simulink library "pbbs_final"  (Simulink 8.1)
settings: Solver=ode1  StartTime=0.0  StopTime=Inf  FixedStep=0.001  RelTol=1e-3
PostLoadFcn:
  | , if any(exist('dsrtsu_mdlpostloadfcn', 'file') == [2, 3, 6]), try dsrtsu_mdlpostloadfcn('Execute', bdroot); catch fprintf('Error in PostLoadFcn (dsrtsu_mdlpostloadfcn) for model "%s":\n %s\n', bdroot, lasterr); end, end,
undefined symbols (not defined in the file or in its folder): KJUD_DecelHardBraking_mps2, KJUD_DecelTGapBraking_s, KJUD_SDFDelay_s, ZERO_FLOAT
libraries: hcu_lib x1, ebdc x1, frdc x1
settings Model: DSRTSU_INTERNAL_RTI_VER=450  DSRTSU_INTERNAL_RTI_TYPE=rti1401  RTICANMMDATA=struct('GeneralSetupData',struct('modelroot','D:\ELN150201\Phase3\branches\ACC_Experiments\AdasDragon\software\sw_development\arch\app\jud','generalsettings',struct('filesettings',struct('destfolder',struct('Name','RTICANMM_FILES','Check',1),'buildfolder',struct('Name','.','Check',1),'AbsDestfolder',struct('Name','D:\ELN150201\Phase3\branches\ACC_Experiments\AdasDragon\software\sw_development\arch\app\jud\RTICANMM_FILES'),'AbsBuildfolder',struct('Name','D:\ELN150201\Phase3\branches\ACC_Experiments\AdasDragon\software\sw_development\arch\app\jud'))),'options',struct('addpaths',1,'rmpaths',1,'addtrcexclusion',logical(1),'cannavigator',struct('checkmonitoring',0),'show_usrtrc',0,'use_usrtrc',0),'advanced',struct('options',[1 1 1 1 1 1 1 1 1 1 1 1 1 1 1 1 1 1 1 1 1 1 1 1 1 1 1 1 1 1 1 1 1 1 1 1 1 1 1 1 1 1 1 1 1 1 1 1 1 1 1 1 1 1 1 1 1 1 1 1 1 1 1 1 1 1 1 1 1 1 1 1 1 1 1 1 1 1 1 1 1 1 1 1 1 1 1 1 1 1 1 1 1 1 1 1 1 1 1 1]),'MPSetup',{{}},'modelname','pbbs_final','block','pbbs_final'))  DSRTSU_INTERNAL_RTIFPGA=40  Creator=tescamilla  LastModifiedBy=AT015555

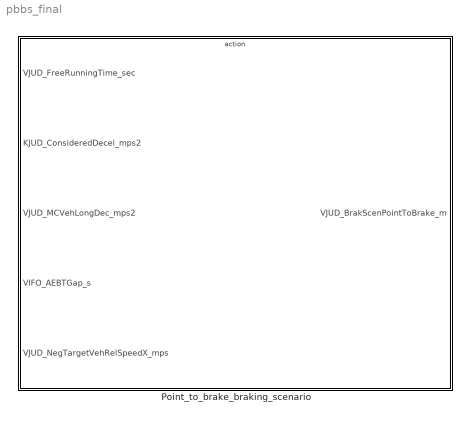
== system pbbs_final ==
  Point_to_brake_braking_scenario : Subsystem

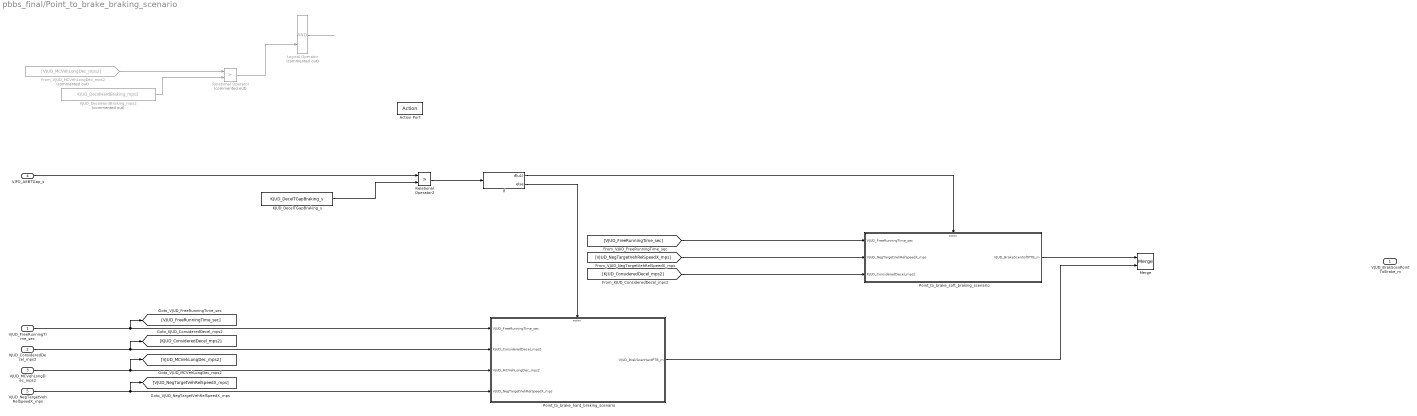
== system pbbs_final/Point_to_brake_braking_scenario ==
  VJUD_FreeRunningTime_sec : Inport
  KJUD_ConsideredDecel_mps2 : Inport  Port=2
  VJUD_MCVehLongDec_mps2 : Inport  Port=3
  VIFO_AEBTGap_s : Inport  Port=4
  VJUD_NegTargetVehRelSpeedX_mps : Inport  Port=5
  Action Port : ActionPort
  From_VJUD_MCVehLongDec_mps2 : From  Commented=on  GotoTag=VJUD_MCVehLongDec_mps2
  If : If  IfExpression=u1
  KJUD_DecelHardBraking_mps2 : Constant  Commented=on  Value=KJUD_DecelHardBraking_mps2  OutDataTypeStr=single
  KJUD_DecelTGapBraking_s : Constant  Value=KJUD_DecelTGapBraking_s  OutDataTypeStr=single
  Logical Operator : Logic  Commented=on  AllPortsSameDT=off  OutDataTypeStr=boolean
  Merge : Merge
  Point_to_brake_hard_braking_scenario : Subsystem  TreatAsAtomicUnit=on
  Point_to_brake_soft_braking_scenario : Subsystem
  Relational Operator : RelationalOperator  Commented=on  Operator=>  OutDataTypeStr=boolean
  Relational Operator2 : RelationalOperator  Operator=>  OutDataTypeStr=boolean
  VJUD_BrakScenPointToBrake_m : Outport
  wires:
  ? -> VJUD_BrakScenPointToBrake_m/1  "VJUD_BrakScenPointToBrake_m"
  [VJUD_NegTargetVehRelSpeedX_mps] -> Point_to_brake_soft_braking_scenario/2(VJUD_NegTargetVehRelSpeedX_mps)
  [KJUD_ConsideredDecel_mps2] -> Point_to_brake_soft_braking_scenario/3(KJUD_ConsideredDecel_mps2)
  [VJUD_FreeRunningTime_sec] -> Point_to_brake_soft_braking_scenario/1(VJUD_FreeRunningTime_sec)
  Point_to_brake_hard_braking_scenario/1(VJUD_BrakScenHardPTB_m) -> Merge/2
  Point_to_brake_soft_braking_scenario/1(VJUD_BrakeScenSoftPTB_m) -> Merge/1
  VJUD_MCVehLongDec_mps2/1 -> Point_to_brake_hard_braking_scenario/3(VJUD_MCVehLongDec_mps2), [VJUD_MCVehLongDec_mps2]
  VJUD_FreeRunningTime_sec/1 -> Point_to_brake_hard_braking_scenario/1(VJUD_FreeRunningTime_sec), [VJUD_FreeRunningTime_sec]
  KJUD_ConsideredDecel_mps2/1 -> [KJUD_ConsideredDecel_mps2], Point_to_brake_hard_braking_scenario/2(KJUD_ConsideredDecel_mps2)
  VJUD_NegTargetVehRelSpeedX_mps/1 -> Point_to_brake_hard_braking_scenario/4(VJUD_NegTargetVehRelSpeedX_mps), [VJUD_NegTargetVehRelSpeedX_mps]
  If/2 -> Point_to_brake_hard_braking_scenario/Action
  If/1 -> Point_to_brake_soft_braking_scenario/Action
  Logical Operator/1 -> ?
  Relational Operator/1 -> Logical Operator/2
  KJUD_DecelHardBraking_mps2/1 -> Relational Operator/2
  From_VJUD_MCVehLongDec_mps2/1 -> Relational Operator/1
  Relational Operator2/1 -> If/1
  VIFO_AEBTGap_s/1 -> Relational Operator2/1
  KJUD_DecelTGapBraking_s/1 -> Relational Operator2/2

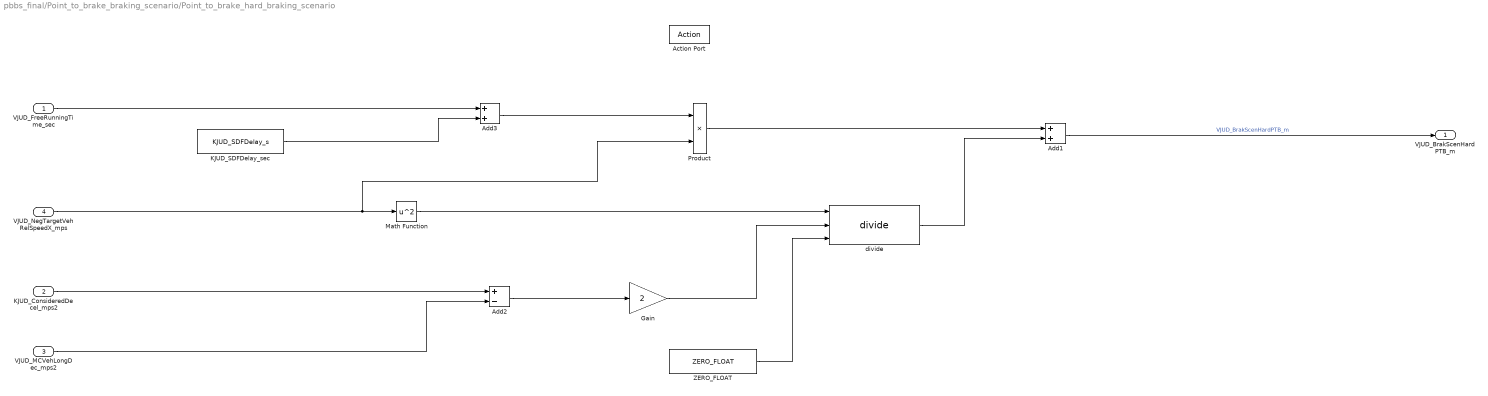
== system pbbs_final/Point_to_brake_braking_scenario/Point_to_brake_hard_braking_scenario ==
  VJUD_FreeRunningTime_sec : Inport
  KJUD_ConsideredDecel_mps2 : Inport  Port=2
  VJUD_MCVehLongDec_mps2 : Inport  Port=3
  VJUD_NegTargetVehRelSpeedX_mps : Inport  Port=4
  Action Port : ActionPort
  Add1 : Sum
  Add2 : Sum  Inputs=+-
  Add3 : Sum
  Gain : Gain  Gain=2
  KJUD_SDFDelay_sec : Constant  Value=KJUD_SDFDelay_s
  Math Function : Math  Operator=square  SaturateOnIntegerOverflow=on
  Product : Product
  ZERO_FLOAT : Constant  Value=ZERO_FLOAT
  divide : hcu_lib/divide
  VJUD_BrakScenHardPTB_m : Outport
  wires:
  KJUD_SDFDelay_sec/1 -> Add3/2
  Add3/1 -> Product/1
  KJUD_ConsideredDecel_mps2/1 -> Add2/1
  Add2/1 -> Gain/1
  ZERO_FLOAT/1 -> divide/3
  Math Function/1 -> divide/1
  VJUD_MCVehLongDec_mps2/1 -> Add2/2
  divide/1 -> Add1/2
  Product/1 -> Add1/1
  Gain/1 -> divide/2
  VJUD_NegTargetVehRelSpeedX_mps/1 -> Math Function/1, Product/2
  Add1/1 -> VJUD_BrakScenHardPTB_m/1  "VJUD_BrakScenHardPTB_m"
  VJUD_FreeRunningTime_sec/1 -> Add3/1

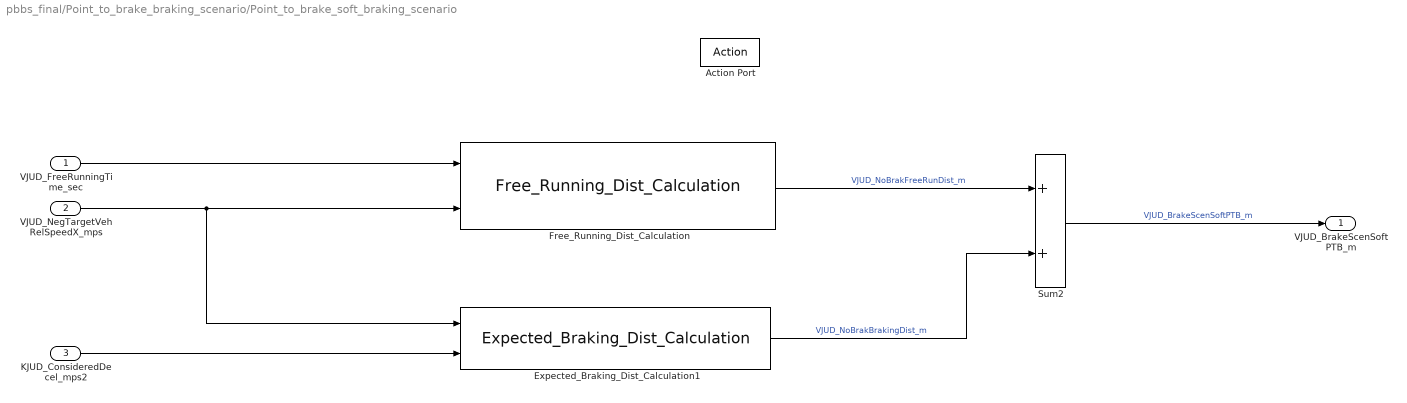
== system pbbs_final/Point_to_brake_braking_scenario/Point_to_brake_soft_braking_scenario ==
  VJUD_FreeRunningTime_sec : Inport
  VJUD_NegTargetVehRelSpeedX_mps : Inport  Port=2
  KJUD_ConsideredDecel_mps2 : Inport  Port=3
  Action Port : ActionPort
  Expected_Braking_Dist_Calculation1 : ebdc/Expected_Braking_Dist_Calculation
  Free_Running_Dist_Calculation : frdc/Free_Running_Dist_Calculation
  Sum2 : Sum
  VJUD_BrakeScenSoftPTB_m : Outport
  wires:
  VJUD_FreeRunningTime_sec/1 -> Free_Running_Dist_Calculation/1
  Sum2/1 -> VJUD_BrakeScenSoftPTB_m/1  "VJUD_BrakeScenSoftPTB_m"
  Expected_Braking_Dist_Calculation1/1 -> Sum2/2  "VJUD_NoBrakBrakingDist_m"
  KJUD_ConsideredDecel_mps2/1 -> Expected_Braking_Dist_Calculation1/2
  Free_Running_Dist_Calculation/1 -> Sum2/1  "VJUD_NoBrakFreeRunDist_m"
  VJUD_NegTargetVehRelSpeedX_mps/1 -> Free_Running_Dist_Calculation/2, Expected_Braking_Dist_Calculation1/1
